simulink library "OUT"  (R2024b)
settings: Solver=VariableStepAuto  StartTime=0.0  StopTime=10.0  RelTol=1e-3
libraries: simulink x1
settings Model: Creator=blatak  LastModifiedBy=blatak
settings ModelReferenceCC: EnableRefExpFcnMdlSchedulingChecks=on
settings RTWCC: GPUComputeCapability=3.5

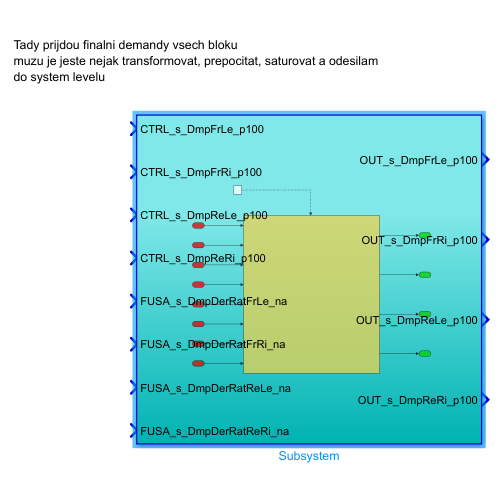
[thumbnail: Simulink's stored preview of the top-level diagram]
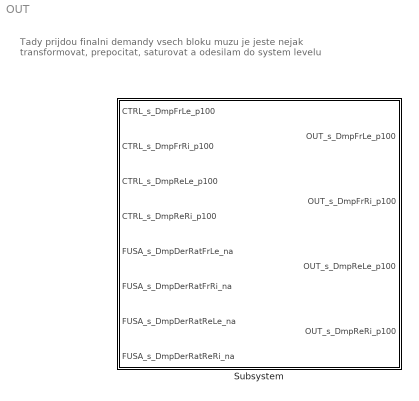
== system OUT ==
  note: Tady prijdou finalni demandy vsech bloku
      | muzu je jeste nejak transformovat, prepocitat, saturovat a odesilam
      | do system levelu
  Subsystem : Subsystem

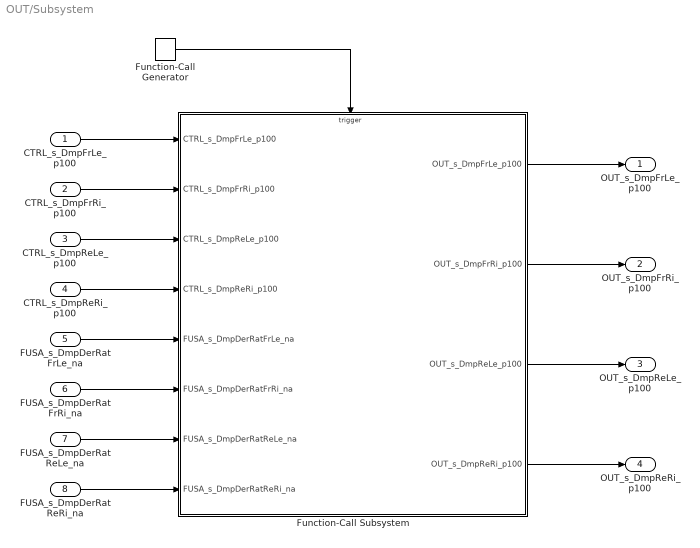
== system OUT/Subsystem ==
  CTRL_s_DmpFrLe_p100 : Inport
  CTRL_s_DmpFrRi_p100 : Inport  Port=2
  CTRL_s_DmpReLe_p100 : Inport  Port=3
  CTRL_s_DmpReRi_p100 : Inport  Port=4
  FUSA_s_DmpDerRatFrLe_na : Inport  Port=5
  FUSA_s_DmpDerRatFrRi_na : Inport  Port=6
  FUSA_s_DmpDerRatReLe_na : Inport  Port=7
  FUSA_s_DmpDerRatReRi_na : Inport  Port=8
  Function-Call Generator : simulink/Ports & Subsystems/Function-Call Generator  sample_time=0.005  numberOfIterations=1  DisallowWideOutput=off
  Function-Call Subsystem : Subsystem  TreatAsAtomicUnit=on
  OUT_s_DmpFrLe_p100 : Outport
  OUT_s_DmpFrRi_p100 : Outport  Port=2
  OUT_s_DmpReLe_p100 : Outport  Port=3
  OUT_s_DmpReRi_p100 : Outport  Port=4
  wires:
  Function-Call Generator/1 -> Function-Call Subsystem/Trigger
  CTRL_s_DmpFrLe_p100/1 -> Function-Call Subsystem/1(CTRL_s_DmpFrLe_p100)
  Function-Call Subsystem/1(OUT_s_DmpFrLe_p100) -> OUT_s_DmpFrLe_p100/1
  Function-Call Subsystem/2(OUT_s_DmpFrRi_p100) -> OUT_s_DmpFrRi_p100/1
  Function-Call Subsystem/3(OUT_s_DmpReLe_p100) -> OUT_s_DmpReLe_p100/1
  Function-Call Subsystem/4(OUT_s_DmpReRi_p100) -> OUT_s_DmpReRi_p100/1
  CTRL_s_DmpFrRi_p100/1 -> Function-Call Subsystem/2(CTRL_s_DmpFrRi_p100)
  CTRL_s_DmpReLe_p100/1 -> Function-Call Subsystem/3(CTRL_s_DmpReLe_p100)
  CTRL_s_DmpReRi_p100/1 -> Function-Call Subsystem/4(CTRL_s_DmpReRi_p100)
  FUSA_s_DmpDerRatFrLe_na/1 -> Function-Call Subsystem/5(FUSA_s_DmpDerRatFrLe_na)
  FUSA_s_DmpDerRatFrRi_na/1 -> Function-Call Subsystem/6(FUSA_s_DmpDerRatFrRi_na)
  FUSA_s_DmpDerRatReLe_na/1 -> Function-Call Subsystem/7(FUSA_s_DmpDerRatReLe_na)
  FUSA_s_DmpDerRatReRi_na/1 -> Function-Call Subsystem/8(FUSA_s_DmpDerRatReRi_na)

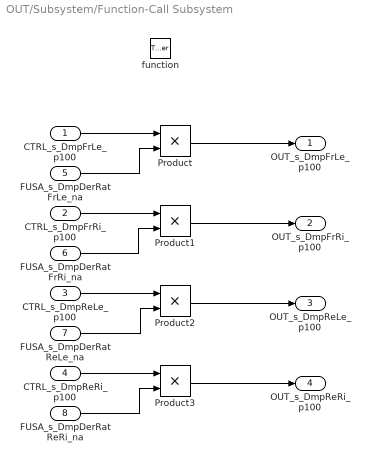
== system OUT/Subsystem/Function-Call Subsystem ==
  CTRL_s_DmpFrLe_p100 : Inport
  CTRL_s_DmpFrRi_p100 : Inport  Port=2
  CTRL_s_DmpReLe_p100 : Inport  Port=3
  CTRL_s_DmpReRi_p100 : Inport  Port=4
  FUSA_s_DmpDerRatFrLe_na : Inport  Port=5
  FUSA_s_DmpDerRatFrRi_na : Inport  Port=6
  FUSA_s_DmpDerRatReLe_na : Inport  Port=7
  FUSA_s_DmpDerRatReRi_na : Inport  Port=8
  function : TriggerPort  TriggerType=function-call  VariantControl=(inherit)
  Product{,1..3} (4 alike) : Product
  OUT_s_DmpFrLe_p100 : Outport
  OUT_s_DmpFrRi_p100 : Outport  Port=2
  OUT_s_DmpReLe_p100 : Outport  Port=3
  OUT_s_DmpReRi_p100 : Outport  Port=4
  wires:
  CTRL_s_DmpFrLe_p100/1 -> Product/1
  FUSA_s_DmpDerRatFrLe_na/1 -> Product/2
  Product/1 -> OUT_s_DmpFrLe_p100/1
  CTRL_s_DmpFrRi_p100/1 -> Product1/1
  FUSA_s_DmpDerRatFrRi_na/1 -> Product1/2
  Product1/1 -> OUT_s_DmpFrRi_p100/1
  CTRL_s_DmpReLe_p100/1 -> Product2/1
  FUSA_s_DmpDerRatReLe_na/1 -> Product2/2
  Product2/1 -> OUT_s_DmpReLe_p100/1
  CTRL_s_DmpReRi_p100/1 -> Product3/1
  FUSA_s_DmpDerRatReRi_na/1 -> Product3/2
  Product3/1 -> OUT_s_DmpReRi_p100/1
